simulink model "B_11"  (R2018b)
settings: Solver=FixedStepDiscrete  StartTime=0.0  StopTime=0.05  MaxStep=1e-4  RelTol=1e-6
StopFcn:
  | %CELEC_plot;
libraries: powerlib x7, simulink x5, peGeneralControl x2
settings Model: Creator=Administrator  LastModifiedBy=Administrator

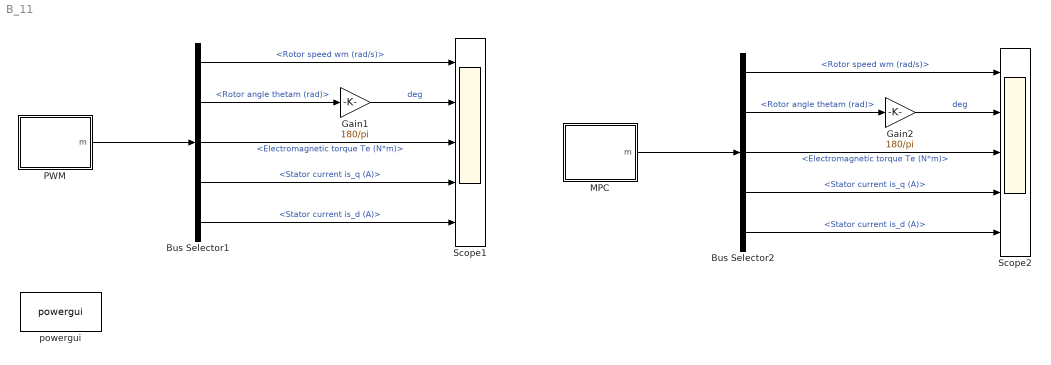
== system B_11 ==
  Bus Selector1 : BusSelector  OutputSignals=Rotor speed wm (rad/s),Rotor angle thetam (rad),Electromagnetic torque Te (N*m),Stator current is_q (A),Stator current is_d (A)
  Bus Selector2 : BusSelector  OutputSignals=Rotor speed wm (rad/s),Rotor angle thetam (rad),Electromagnetic torque Te (N*m),Stator current is_q (A),Stator current is_d (A)
  Gain1 : Gain  Gain=180/pi
  Gain2 : Gain  Gain=180/pi
  MPC : Subsystem  mask{Va=20/sqrt(3), Vb=0, Vc=-20/sqrt(3), t0=0}
  PWM : Subsystem  mask{Va=20/sqrt(3), Vb=0, Vc=-20/sqrt(3), t0=0}
  Scope1 : Scope  NumInputPorts=5
  Scope2 : Scope  NumInputPorts=5
  powergui : powerlib/powergui  Priority=1  SimulationMode=Discrete  SampleTime=2e-6  frequency=60  Iterations=50  frequencyindice=0  Pbase=100e6  ErrMax=1e-4  UnitsV=kV  UnitsW=MW  buscounter=0  FunctionMessages=off  echomessages=off  EnableUseOfTLC=off  CurrentSourceSwitches=off  DisableSnubberDevices=off  DisableRonSwitches=off  DisableVfSwitches=off  DisplayEquations=off  SolverType=Tustin/Backward Euler (TBE)  Interpol=off  ExternalGateDelay=off  methode=off  Ts=100  x0status=blocks  SPID=on  SwTol=0  HookPort=off  RestoreLinks=warning  ResistiveCurrentMeasurement=off  Frange=[0:2:500]  Ylog=off  Xlog=on  ShowGrid=off  save=off  variable=ZData  structure=0  ZoomFFT=off  StartTime=0.0  cycles=1  DisplayStyle=1  fundamental=60  FreqAxis=off  MaxFrequency=1000  frequencyindicesteady=1  RmsSteady=1  display=off
  wires:
  Gain1/1 -> Scope1/2  "deg"
  Bus Selector1/3 -> Scope1/3  "<Electromagnetic torque Te (N*m)>"
  Bus Selector1/4 -> Scope1/4  "<Stator current is_q (A)>"
  PWM/1(m) -> Bus Selector1/1
  Bus Selector1/5 -> Scope1/5  "<Stator current is_d (A)>"
  Bus Selector1/1 -> Scope1/1  "<Rotor speed wm (rad/s)>"
  Bus Selector1/2 -> Gain1/1  "<Rotor angle thetam (rad)>"
  Bus Selector2/1 -> Scope2/1  "<Rotor speed wm (rad/s)>"
  Bus Selector2/3 -> Scope2/3  "<Electromagnetic torque Te (N*m)>"
  Bus Selector2/2 -> Gain2/1  "<Rotor angle thetam (rad)>"
  MPC/1(m) -> Bus Selector2/1
  Bus Selector2/4 -> Scope2/4  "<Stator current is_q (A)>"
  Gain2/1 -> Scope2/2  "deg"
  Bus Selector2/5 -> Scope2/5  "<Stator current is_d (A)>"

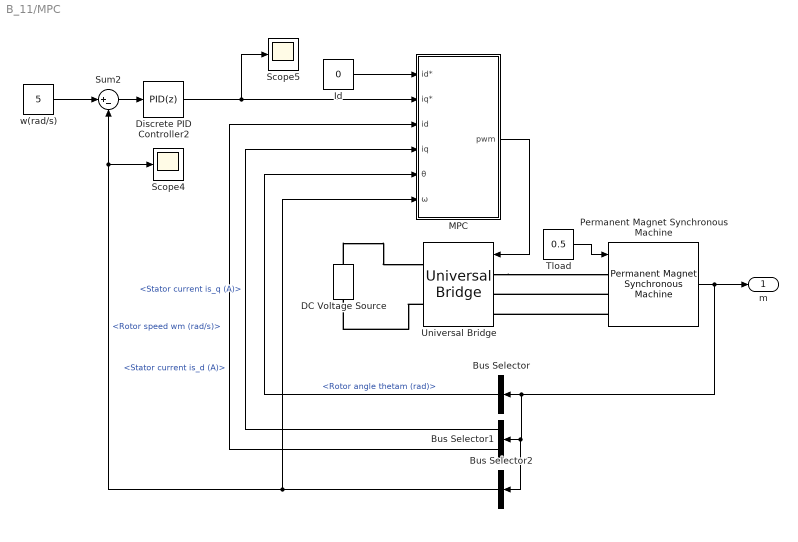
== system B_11/MPC ==
  Bus Selector : BusSelector  OutputSignals=Rotor angle thetam (rad)
  Bus Selector1 : BusSelector  OutputSignals=Stator current is_q (A),Stator current is_d (A)
  Bus Selector2 : BusSelector  OutputSignals=Rotor speed wm (rad/s)
  DC Voltage Source : powerlib/Electrical Sources/DC Voltage Source  Amplitude=100  Measurements=None
  Discrete PID Controller2 : simulink/Continuous/PID Controller  Controller=PID  Form=Parallel  TimeDomain=Discrete-time  SampleTime=-1  IntegratorMethod=Forward Euler  FilterMethod=Forward Euler  ControllerParametersSource=internal  P=20  I=500  D=0  UseFilter=on  N=100  TunerSelectOption=Transfer Function Based (PID Tuner App)  InitialConditionSource=internal  InitialConditionForIntegrator=0  InitialConditionForFilter=0  DifferentiatorICPrevScaledInput=0  ExternalReset=none  TrackingMode=off  Kt=1  LimitOutput=on  UpperSaturationLimit=100  LowerSaturationLimit=-100  LinearizeAsGain=off  AntiWindupMode=none  Kb=1  POutMin=[]  POutMax=[]  IOutMin=[]  IOutMax=[]  DOutMin=[]  DOutMax=[]  NOutMin=[]  NOutMax=[]  SumOutMin=[]  SumOutMax=[]  SaturationOutMin=[]  SaturationOutMax=[]  PParamMin=[]  PParamMax=[]  IParamMin=[]  IParamMax=[]  DParamMin=[]  DParamMax=[]  NParamMin=[]  NParamMax=[]  KbParamMin=[]  KbParamMax=[]  KtParamMin=[]  KtParamMax=[]  KbOutMin=[]  KbOutMax=[]  KtOutMin=[]  KtOutMax=[]  IntegratorOutMin=[]  IntegratorOutMax=[]  FilterOutMin=[]  FilterOutMax=[]  SumI1OutMin=[]  SumI1OutMax=[]  SumI2OutMin=[]  SumI2OutMax=[]  SumI3OutMin=[]  SumI3OutMax=[]  SumI4OutMin=[]  SumI4OutMax=[]  SumDOutMin=[]  SumDOutMax=[]  DifferentiatorOutMin=[]  DifferentiatorOutMax=[]  FilterDiffOutCoefMin=[]  FilterDiffOutCoefMax=[]  ReciprocalOutMin=[]  ReciprocalOutMax=[]  SumDenOutMin=[]  SumDenOutMax=[]  SumNumOutMin=[]  SumNumOutMax=[]  DivideOutMin=[]  DivideOutMax=[]  IntegratorContinuousStateAttributes=''  IntegratorStateMustResolveToSignalObject=off  IntegratorRTWStateStorageClass=Auto  FilterContinuousStateAttributes=''  FilterStateMustResolveToSignalObject=off  FilterRTWStateStorageClass=Auto  ParallelPVariant=InternalParameters  IdealPVariant=Disabled  IVariant=InternalParameters  DVariant=InternalParameters  IntegratorVariant=Discrete  SatVariant=Enabled  AWVariant=Passthrough  PCopyVariant=Disabled  TRVariant=Disabled  FdbkBlocksVariant=Forward  IdealPFdbkVariant=Disabled  SatFdbkVariant=Disabled  DerivativeFilterVariant=ForwardEulerFilter  NVariant=InternalParameters  NCopyVariant=Disabled  FilterICVariant=InternalICsFilter  IntegratorICVariant=InternalICs  ExternalResetVariant=Disabled  TRSumVariant=Passthrough  SumFdbkVariant=Disabled  SumVariant=Sum_PID
  Id : Constant  Value=0
  MPC : Subsystem  mask{Vdc=100, R=0.0485, Ld=0.000395, Lq=0.000395, Phif=0.1194}
      mask prompts: Vdc "直流电压Vdc(V)"; R "R(Ω)"; Ld "Ld(H)"; Lq "Lq(H)"; Phif "ψf(Wb)"
  Permanent Magnet Synchronous Machine : powerlib/Machines/Permanent Magnet Synchronous Machine  NbPhases=3  FluxDistribution=Sinusoidal  RotorType=Round  MechanicalLoad=Torque Tm  PresetModel=No  ShowDetailedParameters=on  MeasurementBus=off  Resistance=0.0485  Inductance=8.5e-3  dqInductances=[8.5e-3,8.5e-3]  La=0.000395  MachineConstant=Flux linkage established by magnets (V.s)  Flux=0.1194  VoltageCst=21.6568  TorqueCst=0.1791  Flat=120  Mechanical=[0.0027 0.0624924 1 0]  PolePairs=4  InitialConditions=[0,t0, 0,0]  InitialConditions5ph=[0 0 0 0 0 0]  TsPowergui=0  TsBlock=-1  RefAngle=Aligned with phase A axis (original Park)
      settings: SourceProductName=Simscape Power Systems
  Scope4 : Scope
  Scope5 : Scope
  Sum2 : Sum  Inputs=|+-
  Tload : Constant  Value=0.5
  Universal Bridge : powerlib/Power Electronics/Universal Bridge  Arms=3  SnubberResistance=1e5  SnubberCapacitance=inf  Device=IGBT / Diodes  Ron=1e-3  Lon=0  ForwardVoltages="[  0  0  ]"  ForwardVoltage=0  GTOparameters=[ 10e-6 , 20e-6 ]  IGBTparameters=[ 1e-6 , 2e-6 ]  Measurements=None  Measurements_2=None  converterType=Rectifier
  w(rad/s) : Constant  Value=5
  m : Outport
  wires:
  Tload/1 -> Permanent Magnet Synchronous Machine/1
  Permanent Magnet Synchronous Machine/1 -> Bus Selector2/1, Bus Selector1/1, Bus Selector/1, m/1
  Discrete PID Controller2/1 -> Scope5/1, MPC/2(iq*)
  Bus Selector1/1 -> MPC/4(iq)  "<Stator current is_q (A)>"
  Bus Selector1/2 -> MPC/3(id)  "<Stator current is_d (A)>"
  Sum2/1 -> Discrete PID Controller2/1
  w(rad/s)/1 -> Sum2/1
  Bus Selector2/1 -> Scope4/1, Sum2/2, MPC/6(ω)  "<Rotor speed wm (rad/s)>"
  Id/1 -> MPC/1(id*)
  Bus Selector/1 -> MPC/5(θ)  "<Rotor angle thetam (rad)>"
  MPC/1(pwm) -> Universal Bridge/1
  connections:
  Permanent Magnet Synchronous Machine/LConn3 -- Universal Bridge/LConn3
  Universal Bridge/LConn1 -- Permanent Magnet Synchronous Machine/LConn1
  Permanent Magnet Synchronous Machine/LConn2 -- Universal Bridge/LConn2
  DC Voltage Source/RConn1 -- Universal Bridge/RConn1
  Universal Bridge/RConn2 -- DC Voltage Source/LConn1

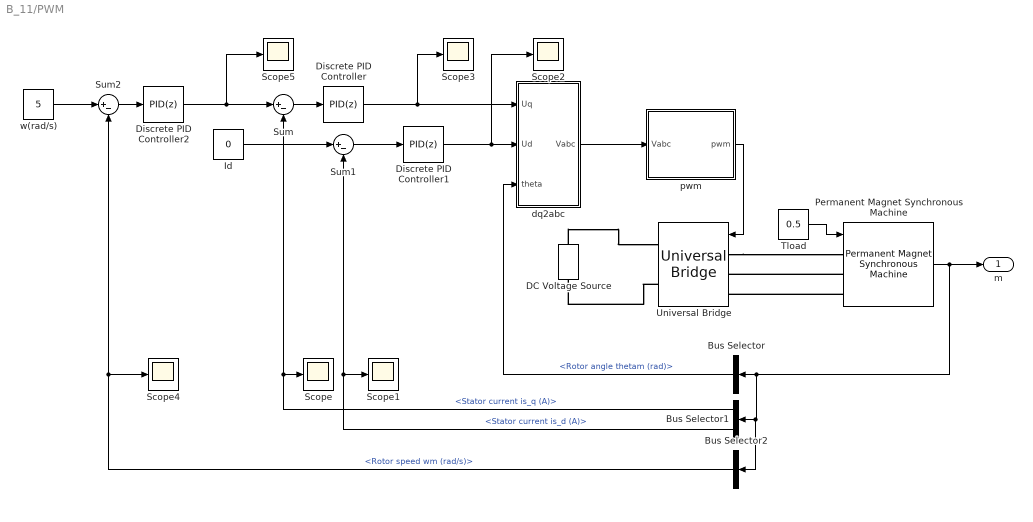
== system B_11/PWM ==
  Bus Selector : BusSelector  OutputSignals=Rotor angle thetam (rad)
  Bus Selector1 : BusSelector  OutputSignals=Stator current is_q (A),Stator current is_d (A)
  Bus Selector2 : BusSelector  OutputSignals=Rotor speed wm (rad/s)
  DC Voltage Source : powerlib/Electrical Sources/DC Voltage Source  Amplitude=100  Measurements=None
  Discrete PID Controller : simulink/Continuous/PID Controller  Controller=PID  Form=Parallel  TimeDomain=Discrete-time  SampleTime=-1  IntegratorMethod=Forward Euler  FilterMethod=Forward Euler  ControllerParametersSource=internal  P=50  I=5000  D=0  UseFilter=on  N=100  TunerSelectOption=Transfer Function Based (PID Tuner App)  InitialConditionSource=internal  InitialConditionForIntegrator=0  InitialConditionForFilter=0  DifferentiatorICPrevScaledInput=0  ExternalReset=none  TrackingMode=off  Kt=1  LimitOutput=on  UpperSaturationLimit=100  LowerSaturationLimit=-100  LinearizeAsGain=off  AntiWindupMode=none  Kb=1  POutMin=[]  POutMax=[]  IOutMin=[]  IOutMax=[]  DOutMin=[]  DOutMax=[]  NOutMin=[]  NOutMax=[]  SumOutMin=[]  SumOutMax=[]  SaturationOutMin=[]  SaturationOutMax=[]  PParamMin=[]  PParamMax=[]  IParamMin=[]  IParamMax=[]  DParamMin=[]  DParamMax=[]  NParamMin=[]  NParamMax=[]  KbParamMin=[]  KbParamMax=[]  KtParamMin=[]  KtParamMax=[]  KbOutMin=[]  KbOutMax=[]  KtOutMin=[]  KtOutMax=[]  IntegratorOutMin=[]  IntegratorOutMax=[]  FilterOutMin=[]  FilterOutMax=[]  SumI1OutMin=[]  SumI1OutMax=[]  SumI2OutMin=[]  SumI2OutMax=[]  SumI3OutMin=[]  SumI3OutMax=[]  SumI4OutMin=[]  SumI4OutMax=[]  SumDOutMin=[]  SumDOutMax=[]  DifferentiatorOutMin=[]  DifferentiatorOutMax=[]  FilterDiffOutCoefMin=[]  FilterDiffOutCoefMax=[]  ReciprocalOutMin=[]  ReciprocalOutMax=[]  SumDenOutMin=[]  SumDenOutMax=[]  SumNumOutMin=[]  SumNumOutMax=[]  DivideOutMin=[]  DivideOutMax=[]  IntegratorContinuousStateAttributes=''  IntegratorStateMustResolveToSignalObject=off  IntegratorRTWStateStorageClass=Auto  FilterContinuousStateAttributes=''  FilterStateMustResolveToSignalObject=off  FilterRTWStateStorageClass=Auto  ParallelPVariant=InternalParameters  IdealPVariant=Disabled  IVariant=InternalParameters  DVariant=InternalParameters  IntegratorVariant=Discrete  SatVariant=Enabled  AWVariant=Passthrough  PCopyVariant=Disabled  TRVariant=Disabled  FdbkBlocksVariant=Forward  IdealPFdbkVariant=Disabled  SatFdbkVariant=Disabled  DerivativeFilterVariant=ForwardEulerFilter  NVariant=InternalParameters  NCopyVariant=Disabled  FilterICVariant=InternalICsFilter  IntegratorICVariant=InternalICs  ExternalResetVariant=Disabled  TRSumVariant=Passthrough  SumFdbkVariant=Disabled  SumVariant=Sum_PID
  Discrete PID Controller1 : simulink/Continuous/PID Controller  Controller=PID  Form=Parallel  TimeDomain=Discrete-time  SampleTime=-1  IntegratorMethod=Forward Euler  FilterMethod=Forward Euler  ControllerParametersSource=internal  P=50  I=5000  D=0  UseFilter=on  N=100  TunerSelectOption=Transfer Function Based (PID Tuner App)  InitialConditionSource=internal  InitialConditionForIntegrator=0  InitialConditionForFilter=0  DifferentiatorICPrevScaledInput=0  ExternalReset=none  TrackingMode=off  Kt=1  LimitOutput=on  UpperSaturationLimit=100  LowerSaturationLimit=-100  LinearizeAsGain=off  AntiWindupMode=none  Kb=1  POutMin=[]  POutMax=[]  IOutMin=[]  IOutMax=[]  DOutMin=[]  DOutMax=[]  NOutMin=[]  NOutMax=[]  SumOutMin=[]  SumOutMax=[]  SaturationOutMin=[]  SaturationOutMax=[]  PParamMin=[]  PParamMax=[]  IParamMin=[]  IParamMax=[]  DParamMin=[]  DParamMax=[]  NParamMin=[]  NParamMax=[]  KbParamMin=[]  KbParamMax=[]  KtParamMin=[]  KtParamMax=[]  KbOutMin=[]  KbOutMax=[]  KtOutMin=[]  KtOutMax=[]  IntegratorOutMin=[]  IntegratorOutMax=[]  FilterOutMin=[]  FilterOutMax=[]  SumI1OutMin=[]  SumI1OutMax=[]  SumI2OutMin=[]  SumI2OutMax=[]  SumI3OutMin=[]  SumI3OutMax=[]  SumI4OutMin=[]  SumI4OutMax=[]  SumDOutMin=[]  SumDOutMax=[]  DifferentiatorOutMin=[]  DifferentiatorOutMax=[]  FilterDiffOutCoefMin=[]  FilterDiffOutCoefMax=[]  ReciprocalOutMin=[]  ReciprocalOutMax=[]  SumDenOutMin=[]  SumDenOutMax=[]  SumNumOutMin=[]  SumNumOutMax=[]  DivideOutMin=[]  DivideOutMax=[]  IntegratorContinuousStateAttributes=''  IntegratorStateMustResolveToSignalObject=off  IntegratorRTWStateStorageClass=Auto  FilterContinuousStateAttributes=''  FilterStateMustResolveToSignalObject=off  FilterRTWStateStorageClass=Auto  ParallelPVariant=InternalParameters  IdealPVariant=Disabled  IVariant=InternalParameters  DVariant=InternalParameters  IntegratorVariant=Discrete  SatVariant=Enabled  AWVariant=Passthrough  PCopyVariant=Disabled  TRVariant=Disabled  FdbkBlocksVariant=Forward  IdealPFdbkVariant=Disabled  SatFdbkVariant=Disabled  DerivativeFilterVariant=ForwardEulerFilter  NVariant=InternalParameters  NCopyVariant=Disabled  FilterICVariant=InternalICsFilter  IntegratorICVariant=InternalICs  ExternalResetVariant=Disabled  TRSumVariant=Passthrough  SumFdbkVariant=Disabled  SumVariant=Sum_PID
  Discrete PID Controller2 : simulink/Continuous/PID Controller  Controller=PID  Form=Parallel  TimeDomain=Discrete-time  SampleTime=-1  IntegratorMethod=Forward Euler  FilterMethod=Forward Euler  ControllerParametersSource=internal  P=20  I=500  D=0  UseFilter=on  N=100  TunerSelectOption=Transfer Function Based (PID Tuner App)  InitialConditionSource=internal  InitialConditionForIntegrator=0  InitialConditionForFilter=0  DifferentiatorICPrevScaledInput=0  ExternalReset=none  TrackingMode=off  Kt=1  LimitOutput=on  UpperSaturationLimit=100  LowerSaturationLimit=-100  LinearizeAsGain=off  AntiWindupMode=none  Kb=1  POutMin=[]  POutMax=[]  IOutMin=[]  IOutMax=[]  DOutMin=[]  DOutMax=[]  NOutMin=[]  NOutMax=[]  SumOutMin=[]  SumOutMax=[]  SaturationOutMin=[]  SaturationOutMax=[]  PParamMin=[]  PParamMax=[]  IParamMin=[]  IParamMax=[]  DParamMin=[]  DParamMax=[]  NParamMin=[]  NParamMax=[]  KbParamMin=[]  KbParamMax=[]  KtParamMin=[]  KtParamMax=[]  KbOutMin=[]  KbOutMax=[]  KtOutMin=[]  KtOutMax=[]  IntegratorOutMin=[]  IntegratorOutMax=[]  FilterOutMin=[]  FilterOutMax=[]  SumI1OutMin=[]  SumI1OutMax=[]  SumI2OutMin=[]  SumI2OutMax=[]  SumI3OutMin=[]  SumI3OutMax=[]  SumI4OutMin=[]  SumI4OutMax=[]  SumDOutMin=[]  SumDOutMax=[]  DifferentiatorOutMin=[]  DifferentiatorOutMax=[]  FilterDiffOutCoefMin=[]  FilterDiffOutCoefMax=[]  ReciprocalOutMin=[]  ReciprocalOutMax=[]  SumDenOutMin=[]  SumDenOutMax=[]  SumNumOutMin=[]  SumNumOutMax=[]  DivideOutMin=[]  DivideOutMax=[]  IntegratorContinuousStateAttributes=''  IntegratorStateMustResolveToSignalObject=off  IntegratorRTWStateStorageClass=Auto  FilterContinuousStateAttributes=''  FilterStateMustResolveToSignalObject=off  FilterRTWStateStorageClass=Auto  ParallelPVariant=InternalParameters  IdealPVariant=Disabled  IVariant=InternalParameters  DVariant=InternalParameters  IntegratorVariant=Discrete  SatVariant=Enabled  AWVariant=Passthrough  PCopyVariant=Disabled  TRVariant=Disabled  FdbkBlocksVariant=Forward  IdealPFdbkVariant=Disabled  SatFdbkVariant=Disabled  DerivativeFilterVariant=ForwardEulerFilter  NVariant=InternalParameters  NCopyVariant=Disabled  FilterICVariant=InternalICsFilter  IntegratorICVariant=InternalICs  ExternalResetVariant=Disabled  TRSumVariant=Passthrough  SumFdbkVariant=Disabled  SumVariant=Sum_PID
  Id : Constant  Value=0
  Permanent Magnet Synchronous Machine : powerlib/Machines/Permanent Magnet Synchronous Machine  NbPhases=3  FluxDistribution=Sinusoidal  RotorType=Round  MechanicalLoad=Torque Tm  PresetModel=No  ShowDetailedParameters=on  MeasurementBus=off  Resistance=0.0485  Inductance=8.5e-3  dqInductances=[8.5e-3,8.5e-3]  La=0.000395  MachineConstant=Flux linkage established by magnets (V.s)  Flux=0.1194  VoltageCst=21.6568  TorqueCst=0.1791  Flat=120  Mechanical=[0.0027 0.0624924 1 0]  PolePairs=4  InitialConditions=[0,t0, 0,0]  InitialConditions5ph=[0 0 0 0 0 0]  TsPowergui=0  TsBlock=-1  RefAngle=Aligned with phase A axis (original Park)
      settings: SourceProductName=Simscape Power Systems
  Scope{,1..5} (6 alike) : Scope
  Sum : Sum  Inputs=|+-
  Sum1 : Sum  Inputs=|+-
  Sum2 : Sum  Inputs=|+-
  Tload : Constant  Value=0.5
  Universal Bridge : powerlib/Power Electronics/Universal Bridge  Arms=3  SnubberResistance=1e5  SnubberCapacitance=inf  Device=IGBT / Diodes  Ron=1e-3  Lon=0  ForwardVoltages="[  0  0  ]"  ForwardVoltage=0  GTOparameters=[ 10e-6 , 20e-6 ]  IGBTparameters=[ 1e-6 , 2e-6 ]  Measurements=None  Measurements_2=None  converterType=Rectifier
  dq2abc : Subsystem
  pwm : Subsystem
  w(rad/s) : Constant  Value=5
  m : Outport
  wires:
  Tload/1 -> Permanent Magnet Synchronous Machine/1
  Permanent Magnet Synchronous Machine/1 -> Bus Selector2/1, Bus Selector1/1, Bus Selector/1, m/1
  Discrete PID Controller2/1 -> Scope5/1, Sum/1
  Discrete PID Controller1/1 -> Scope2/1, dq2abc/2(Ud)
  Bus Selector/1 -> dq2abc/3(theta)  "<Rotor angle thetam (rad)>"
  Sum/1 -> Discrete PID Controller/1
  Discrete PID Controller/1 -> Scope3/1, dq2abc/1(Uq)
  Id/1 -> Sum1/1
  Sum1/1 -> Discrete PID Controller1/1
  Bus Selector1/1 -> Scope/1, Sum/2  "<Stator current is_q (A)>"
  Bus Selector1/2 -> Scope1/1, Sum1/2  "<Stator current is_d (A)>"
  Sum2/1 -> Discrete PID Controller2/1
  w(rad/s)/1 -> Sum2/1
  Bus Selector2/1 -> Scope4/1, Sum2/2  "<Rotor speed wm (rad/s)>"
  dq2abc/1(Vabc) -> pwm/1(Vabc)
  pwm/1(pwm) -> Universal Bridge/1
  connections:
  Permanent Magnet Synchronous Machine/LConn3 -- Universal Bridge/LConn3
  Universal Bridge/LConn1 -- Permanent Magnet Synchronous Machine/LConn1
  Permanent Magnet Synchronous Machine/LConn2 -- Universal Bridge/LConn2
  DC Voltage Source/RConn1 -- Universal Bridge/RConn1
  Universal Bridge/RConn2 -- DC Voltage Source/LConn1

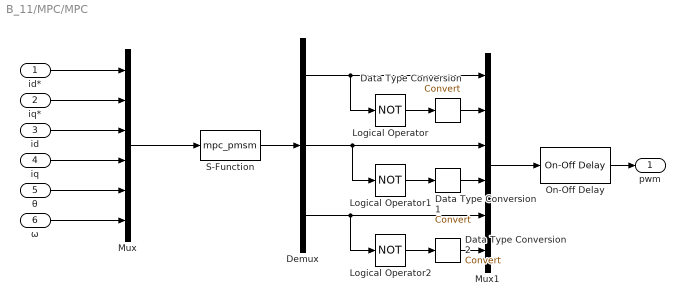
== system B_11/MPC/MPC ==
  id* : Inport
  iq* : Inport  Port=2
  id : Inport  Port=3
  iq : Inport  Port=4
  θ : Inport  Port=5
  ω : Inport  Port=6
  Data Type Conversion : DataTypeConversion
  Data Type Conversion1 : DataTypeConversion
  Data Type Conversion2 : DataTypeConversion
  Demux : Demux  Outputs=3
  Logical Operator : Logic  Operator=NOT  AllPortsSameDT=off  OutDataTypeStr=boolean
  Logical Operator1 : Logic  Operator=NOT  AllPortsSameDT=off  OutDataTypeStr=boolean
  Logical Operator2 : Logic  Operator=NOT  AllPortsSameDT=off  OutDataTypeStr=boolean
  Mux : Mux  Inputs=6
  Mux1 : Mux  Inputs=6
  On-Off Delay : peGeneralControl/On-Off Delay  LabelModeActiveChoice=Discrete  Td_on=2e-6  Td_off=0  IC=0  Ts=2e-6
  S-Function : S-Function  FunctionName=mpc_pmsm  Parameters=Vdc,R,Ld,Lq,Phif  SFunctionDeploymentMode=off  EnableBusSupport=off
  pwm : Outport
  wires:
  iq*/1 -> Mux/2
  Mux/1 -> S-Function/1
  S-Function/1 -> Demux/1
  ω/1 -> Mux/6
  id*/1 -> Mux/1
  iq/1 -> Mux/4
  θ/1 -> Mux/5
  id/1 -> Mux/3
  Mux1/1 -> On-Off Delay/1
  On-Off Delay/1 -> pwm/1
  Demux/3 -> Logical Operator2/1, Mux1/5
  Logical Operator1/1 -> Data Type Conversion1/1
  Demux/2 -> Logical Operator1/1, Mux1/3
  Demux/1 -> Logical Operator/1, Mux1/1
  Logical Operator2/1 -> Data Type Conversion2/1
  Logical Operator/1 -> Data Type Conversion/1
  Data Type Conversion/1 -> Mux1/2
  Data Type Conversion1/1 -> Mux1/4
  Data Type Conversion2/1 -> Mux1/6

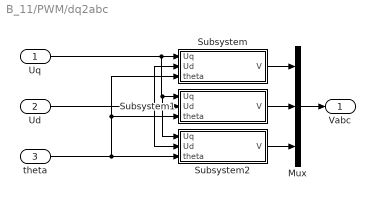
== system B_11/PWM/dq2abc ==
  Uq : Inport
  Ud : Inport  Port=2
  theta : Inport  Port=3
  Mux : Mux  Inputs=3
  Subsystem : Subsystem
  Subsystem1 : Subsystem
  Subsystem2 : Subsystem
  Vabc : Outport
  wires:
  theta/1 -> Subsystem2/3(theta), Subsystem1/3(theta), Subsystem/3(theta)
  Ud/1 -> Subsystem1/2(Ud), Subsystem2/2(Ud), Subsystem/2(Ud)
  Uq/1 -> Subsystem2/1(Uq), Subsystem1/1(Uq), Subsystem/1(Uq)
  Mux/1 -> Vabc/1
  Subsystem/1(V) -> Mux/1
  Subsystem1/1(V) -> Mux/2
  Subsystem2/1(V) -> Mux/3

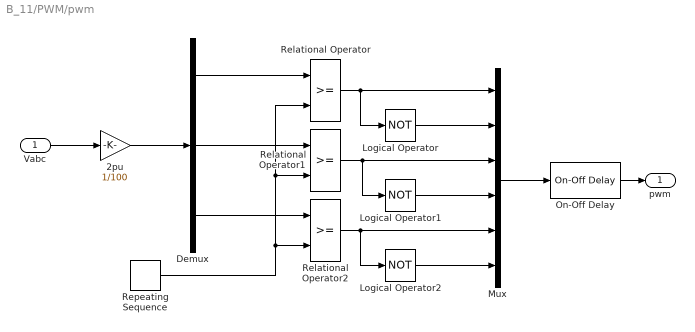
== system B_11/PWM/pwm ==
  Vabc : Inport
  2pu : Gain  Gain=1/100
  Demux : Demux  Outputs=3
  Logical Operator : Logic  Operator=NOT  AllPortsSameDT=off  OutDataTypeStr=boolean
  Logical Operator1 : Logic  Operator=NOT  AllPortsSameDT=off  OutDataTypeStr=boolean
  Logical Operator2 : Logic  Operator=NOT  AllPortsSameDT=off  OutDataTypeStr=boolean
  Mux : Mux  Inputs=6
  On-Off Delay : peGeneralControl/On-Off Delay  LabelModeActiveChoice=Discrete  Td_on=2e-6  Td_off=0  IC=0  Ts=2e-6
  Relational Operator : RelationalOperator  OutDataTypeStr=boolean  RndMeth=Simplest
  Relational Operator1 : RelationalOperator  OutDataTypeStr=boolean  RndMeth=Simplest
  Relational Operator2 : RelationalOperator  OutDataTypeStr=boolean  RndMeth=Simplest
  Repeating Sequence : simulink/Sources/Repeating Sequence  rep_seq_t=[0 0.0001]  rep_seq_y=[-1 1]
  pwm : Outport
  wires:
  Repeating Sequence/1 -> Relational Operator2/2, Relational Operator1/2, Relational Operator/2
  Demux/1 -> Relational Operator/1
  Logical Operator/1 -> Mux/2
  Relational Operator/1 -> Mux/1, Logical Operator/1
  Relational Operator1/1 -> Logical Operator1/1, Mux/3
  Logical Operator1/1 -> Mux/4
  Relational Operator2/1 -> Logical Operator2/1, Mux/5
  Logical Operator2/1 -> Mux/6
  Mux/1 -> On-Off Delay/1
  Demux/2 -> Relational Operator1/1
  Demux/3 -> Relational Operator2/1
  Vabc/1 -> 2pu/1
  2pu/1 -> Demux/1
  On-Off Delay/1 -> pwm/1

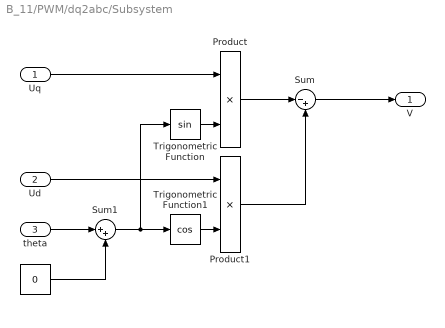
== system B_11/PWM/dq2abc/Subsystem ==
  Uq : Inport
  Ud : Inport  Port=2
  theta : Inport  Port=3
  "  " : Constant  Value=0
  Product : Product
  Product1 : Product
  Sum : Sum  Inputs=|-+
  Sum1 : Sum  Inputs=|++
  Trigonometric Function : Trigonometry
  Trigonometric Function1 : Trigonometry  Operator=cos
  V : Outport
  wires:
  Trigonometric Function1/1 -> Product1/2
  Sum1/1 -> Trigonometric Function/1, Trigonometric Function1/1
  Sum/1 -> V/1
  Trigonometric Function/1 -> Product/2
  Uq/1 -> Product/1
  Product/1 -> Sum/1
  Product1/1 -> Sum/2
  Ud/1 -> Product1/1
  theta/1 -> Sum1/1
  "  "/1 -> Sum1/2

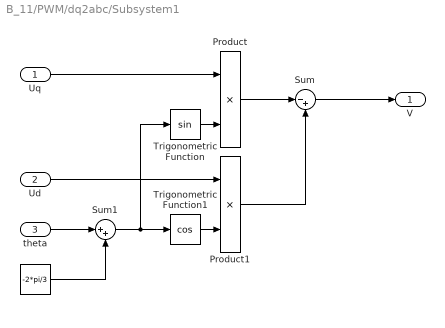
== system B_11/PWM/dq2abc/Subsystem1 ==
  Uq : Inport
  Ud : Inport  Port=2
  theta : Inport  Port=3
  "  " : Constant  Value=-2*pi/3
  Product : Product
  Product1 : Product
  Sum : Sum  Inputs=|-+
  Sum1 : Sum  Inputs=|++
  Trigonometric Function : Trigonometry
  Trigonometric Function1 : Trigonometry  Operator=cos
  V : Outport
  wires:
  Trigonometric Function1/1 -> Product1/2
  Sum1/1 -> Trigonometric Function/1, Trigonometric Function1/1
  Sum/1 -> V/1
  Trigonometric Function/1 -> Product/2
  Uq/1 -> Product/1
  Product/1 -> Sum/1
  Product1/1 -> Sum/2
  Ud/1 -> Product1/1
  theta/1 -> Sum1/1
  "  "/1 -> Sum1/2

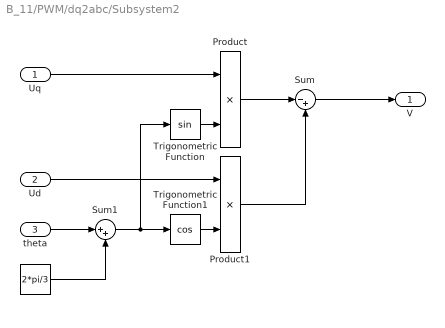
== system B_11/PWM/dq2abc/Subsystem2 ==
  Uq : Inport
  Ud : Inport  Port=2
  theta : Inport  Port=3
  "  " : Constant  Value=2*pi/3
  Product : Product
  Product1 : Product
  Sum : Sum  Inputs=|-+
  Sum1 : Sum  Inputs=|++
  Trigonometric Function : Trigonometry
  Trigonometric Function1 : Trigonometry  Operator=cos
  V : Outport
  wires:
  Trigonometric Function1/1 -> Product1/2
  Sum1/1 -> Trigonometric Function/1, Trigonometric Function1/1
  Sum/1 -> V/1
  Trigonometric Function/1 -> Product/2
  Uq/1 -> Product/1
  Product/1 -> Sum/1
  Product1/1 -> Sum/2
  Ud/1 -> Product1/1
  theta/1 -> Sum1/1
  "  "/1 -> Sum1/2
